simulink model "Commande_6_ReglageCascade_LoopShaping"  (R2015a)
settings: Solver=ode45  StartTime=0.0  StopTime=20  RelTol=1e-3
values from neighbouring files (symbols this model uses):
  Kd = p1^2*J4    (= 0.0333)    [A_1_Data.m]    (also in matlab.mat = 0.009)
  Kp = -2*p1*J4    (= 0.00222)    [A_1_Data.m]    (also in matlab.mat = 0.0006)
  s = tf('s')    [A_3_LoopShaping.m]    (also in A_4_Hinfini.m = zpk('s'))
  X = [0;0;0;0;0;0;0;0]    [A_1_Data.m]
  Y = [0;0;0;0;0;0;0;0]    [A_1_Data.m]
undefined symbols (not defined in the file or in its folder): sfun3d, Z
libraries: sm_lib x332, nesl_utility x15, simulink x1
(part 10 of 10)

== matlab function Commande_6_ReglageCascade_LoopShaping/Regulateur de la partie electrique/Calcule de gains1 ==
  data: e input; ei output; ep output
function [ei , ep]= fcn(e)

b1 = -1.1250e+03 ;
Ki=0.119;
% ei  :c'est l'erreur du couple multiplie par le gain de l'integrateur KI(du
% regulateur)
% ei  :c'est l'erreur du couple multiplie par le gain proportinnel Kp (du
% regulateur)

% le pole desire :
p = 2*b1;
Kp= -p/Ki ;
KI = -b1*Kp ;
ep = e*Kp ;
ei = e*KI ;

% Remarque ;
% Ki:constante du couple (couple=Ki*courant)
% KI : pour l'action integrale

== matlab function Commande_6_ReglageCascade_LoopShaping/Trajectoir1/Trajectoir2 ==
  data: t input; ne input; P output; dP output; d2P output; d3P output
function [P,dP,d2P,d3P]= fcn(t,ne)

%% Menu
% 1 ==> Ligne horizontal
% 2==>  Ligne suivant l'axe oz
% 3==> Cercle
% 4==> Ligne x=y
 z0=-0.08789 ; zpi=-0.3;
B= (z0+zpi)/2 ; A= (z0-zpi)/2 ; 
f = 5; f2 = 5 ;
R=0.2;
%% vers le Plan Z=-0.3
if (t<pi/f && (ne == 1 || ne == 3 ||  ne == 0 || ne == 4 || ne == 5 ||  ne == 6))
n= 2 ; 
elseif( (ne == 4 || ne == 5 ||  ne == 6)  &&  (t<3*pi/2/f) ) % vers le point (0 , R , -0.3)
n=1 ;
else
n =ne ;
end

%% le trajecoir
switch n
    
    case 0
        
        % La position
        x = R*sin(f*t)  ; y=0 ;
        z=  zpi ;
        P = [ x ; y ; z ];
        % La vitess
        dx = f*R*cos(f*t)  ; dy=0 ;
        dz= 0 ;
        dP = [ dx ; dy ; dz ];
        % L'acceleration :
        d2x = -f^2*R*sin(f*t) ; d2y=0 ;
        d2z =  0;
        d2P = [ d2x ; d2y ; d2z ];
        % L'a _coup :
        d3x = -f^3*R*cos(f*t) ; d3y=0 ;
        d3z =  0;
        d3P = [ d3x ; d3y ; d3z ];
    case 1   
        % La position
        y = R*sin(f*t)  ; x=0 ;
        z= zpi  ;
        P = [ x ; y ; z ];
        % La vitess
        dy = f*R*cos(f*t)  ; dx=0 ;
        dz= 0 ;
        dP = [ dx ; dy ; dz ];
        % L'acceleration :
        d2y = -f^2*R*sin(f*t) ; d2x=0 ;
        d2z =  0;
        d2P = [ d2x ; d2y ; d2z ];
        % L'a _coup :
        d3y = -f^3*R*cos(f*t) ; d3x=0 ;
        d3z =  0;
        d3P = [ d3x ; d3y ; d3z ];
    case 2
        % La position 
        x = 0 ; y=0 ;
        z= A*cos(f*t) + B ; 
        P = [ x ; y ; z ];
        % La vitess
        dx = 0 ; dy=0 ;
        dz= -f*A*sin(f*t) ;
        dP = [ dx ; dy ; dz ];
        % L'acceleration :
        d2x = 0 ; d2y=0 ;
        d2z = -f^2*A*cos(f*t) ;
        d2P = [ d2x ; d2y ; d2z ];
        % L a_coup (jerk) :
        d3x = 0 ; d3y=0 ;
        d3z = f^3*A*sin(f*t) ;
        d3P = [ d3x ; d3y ; d3z ];
        
        %%
    case 3
        R=0.12;
        y = R*sin(f*t)  ; x=2*y;
        z= zpi  ;
        P = [ x ; y ; z ];
        % La vitess
        dy = f*R*cos(f*t)  ; dx=2*dy ;
        dz= 0 ;
        dP = [ dx ; dy ; dz ];
        % L'acceleration :
        d2y = -f^2*R*sin(f*t) ; d2x=2*d2y ;
        d2z =  0;
        d2P = [ d2x ; d2y ; d2z ];
        % L'a _coup :
        d3y = -f^3*R*cos(f*t) ; d3x=2*d3y ;
        d3z =  0;
        d3P = [ d3x ; d3y ; d3z ];
    case 4 % Cerecl XY
        x=R*cos(f*t) ; y=R*sin(f*t) ; z=zpi  ;
        dx=-f*R*sin(f*t) ; dy=f*R*cos(f*t)  ;  dz=0;
        d2x=-f^2*R*cos(f*t) ; d2y=-f^2*R*sin(f*t)  ;  d2z=0;
        P=[x ; y ; z];
        dP=[dx ; dy ; dz];
        d2P=[d2x ; d2y ; d2z];
        % L'a _coup :
        d3x=f^3*R*sin(f*t) ; d3y=-f^3*R*cos(f*t)  ;  d3z=0;
        d3P=[d3x ; d3y ; d3z];
        
    case 5 % ZY   
        x=0 ; y=R*sin(f*t) ; z=0.5*R*cos(f*t) + zpi  ;
        dx=0 ; dy=f*R*cos(f*t)  ;  dz=-f*0.5*R*sin(f*t);
        d2x=0 ; d2y=-f^2*R*sin(f*t)  ;  d2z=-f^2*0.5*R*cos(f*t);
        P=[x ; y ; z];
        dP=[dx ; dy ; dz];
        d2P=[d2x ; d2y ; d2z];
        d3x=0 ; d3y=-f^3*R*cos(f*t)  ;  d3z=f^3*0.5*R*sin(f*t);
        d3P=[d3x ; d3y ; d3z];
%     case 6 %Cercle ZX
%         y=0 ; x=R*sin(f*t) ; z=R*cos(f*t) +zpi;
%         dy=0 ; dx=f*R*cos(f*t)  ;  dz=-f*R*sin(f*t);
%         d2y=0 ; d2x=-f^2*R*sin(f*t)  ;  d2z=-f^2*R*cos(f*t);
%         d3y=0 ; d3x=-f^3*R*cos(f*t)  ;  d3z=f^3*R*sin(f*t);
%         P=[x ; y ; z];
%         dP=[dx ; dy ; dz];
%         d2P=[d2x ; d2y ; d2z];
%         d3P = [ d3x ; d3y ; d3z ];
%     case 7  % Les derivees sont a corriger
%         R=0.00*sin(f2*t) ; A=0.1270 ;
%         x=R*cos(f*t) ; y=R*sin(f*t) ;
%         z= A*sin(f2*t) -0.2 ;
%         dx=-f*R*sin(f*t) ; dy=f*R*cos(f*t)  ;  
%         dz= f2*A*cos(f2*t) ;
%         d2x=-f^2*R*cos(f*t) ; d2y=-f^2*R*sin(f*t)  ;
%         d2z = -f2^2*A*sin(f2*t) ;
%         P=[x ; y ; z];
%         dP=[dx ; dy ; dz];
%         d2P=[d2x ; d2y ; d2z];
%         % L'a _coup :
%         d3x=f^3*R*sin(f*t) ; d3y=-f^3*R*cos(f*t)  ;
%         d3z = -f2^3*A*cos(f2*t) ;
%         d3P=[d3x ; d3y ; d3z];
    case 8
        x=0 ; y=0 ; z=z0 ;
        P=[x ; y ; z];
        dP=[0 ; 0 ; 0];
        d2P=[0 ; 0 ; 0];
        d3P=[0 ; 0 ; 0];
        
    otherwise
        P=[0 ; 0 ; 0];
        dP=[0 ; 0 ; 0];
        d2P=[0 ; 0 ; 0];
        d3P = [ 0 ; 0 ; 0 ];
end

== matlab function Commande_6_ReglageCascade_LoopShaping/Regulateur de la partie electrique/Decoupleur Tension Vitess ==
  data: DUd input; DU output; DX2 input
function DU = fcn(DUd,DX2)


b2 = -99.4718 ;
b3 =833.3333 ;

DU = (DUd - b2*DX2)/b3 ;
